simulink model "myproject_task"  (Simulink 3.00)
libraries: logiclib x4, mathlib x3, arclib x1

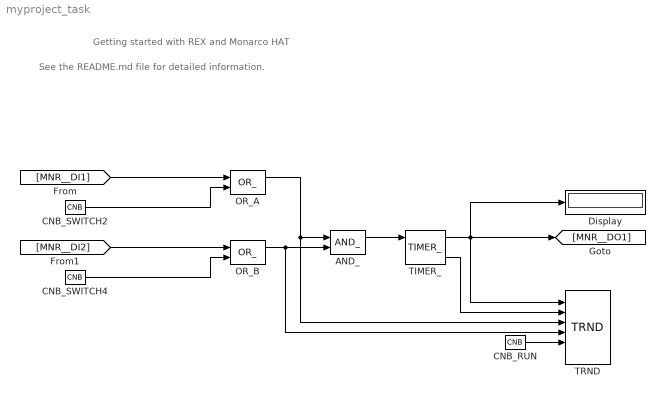
== system myproject_task ==
  note: See the README.md file for detailed information.
  note: Getting started with REX and Monarco HAT
  AND_ : logiclib/AND_
  CNB_RUN : mathlib/CNB  YCN=on
  CNB_SWITCH2 : mathlib/CNB  YCN=off
  CNB_SWITCH4 : mathlib/CNB  YCN=off
  Display : Display
      settings: Format=Best fit
  OR_A : logiclib/OR_
  OR_B : logiclib/OR_
  TIMER_ : logiclib/TIMER_  mode=2: Delayed ON  pt=5
  TRND : arclib/TRND  n=4  l=2000  btype=8: Double  ptype1=1: Store  ptype2=1: Store  ptype3=1: Store  ptype4=1: Store  pfac=1  afac=0  arc=0  id=1  Title=My timer  timesrc=1: CORETIMER
  wires:
  AND_/1 -> TIMER_/1
  CNB_RUN/1 -> TRND/5
  CNB_SWITCH2/1 -> OR_A/2
  CNB_SWITCH4/1 -> OR_B/2
  [MNR__DI1] -> OR_A/1
  [MNR__DI2] -> OR_B/1
  OR_A/1 -> AND_/1, TRND/3
  OR_B/1 -> AND_/2, TRND/4
  TIMER_/1 -> Display/1, [MNR__DO1], TRND/1
  TIMER_/3 -> TRND/2
